simulink model "c6_formation2"  (R2021b)
settings: Solver=FixedStepDiscrete  StartTime=0.0  StopTime=Inf  FixedStep=sampleTime  RelTol=1e-3  EnableMultiTasking=on
PreLoadFcn:
  | %load emptyMap
  | 
  | % Lidar parameters
  | sensorOffset = [0,0];
  | scanAngles = -pi:pi/6:pi;
  | maxRange = 0.25;
InitFcn:
  | sampleTime = 0.05;
  | nMedianSize=3;
  | % Robot parameters
  | wheelRadius = 0.0335;
  | robotRadius = 0.7*0.116;
  | 
  | %角速度坐标
  | ks=1;
  | 
  | % Lidar parameters
  | sensorOffset = [0,0];
  | scanAngles = -pi:pi/36:pi;
  | maxRange = 0.2;
  | 
  | %车初始位置
  | init_pose_1=[1  1.3  pi/2]';
  | init_pose_2=[0.85 1  pi/2]';
  | init_pose_3=[1.15 1  pi/2]';
  | init_pose_4=[0.7  0.7 pi/2]';
  | init_pose_5=[1  0.7 pi/2]';
  | init_pose_6=[1.3 0.7  pi/2]';
  | 
  | %pp算法性能参数
  | Vd_pp=0.25;
  | Wd_pp=0.25*pi;
  | dist_pp=0.2;
  | GoalRadius=0.1;
  | numSector=72;
  | rangeDis=[0.03,maxRange];
  | thresholds=[0.03 0.1];
  | safetyDis=0.1;
  | minimumTurningRadius=0.2*0.2/3;
undefined symbols (not defined in the file): Angular, DiscIntNeverNeededParam, Linear, recovery_w
libraries: robotlib x24, dspstat3 x18, robotalgslib x6
(part 4 of 4)

== matlab function c6_formation2/controller/Car6/ppCar/Compute Velocity and Heading for Path following/Car1/Kinematicc Controller/MATLAB Function ==
  data: psi input; dw output; psid input; x input; xd input; y input; yd input; targetdir output
function [dw,targetdir]= fcn(psi,psid,x,xd,y,yd)

if norm([xd-x,yd-y])<0.15    
    targetdir=angdiff(psi,psid);
    dw=tanh(targetdir);    
else
    dw=0;
    targetdir=angdiff(psi,atan2(yd-y,xd-x));
end

== matlab function c6_formation2/controller/controller1/MATLAB Function5 ==
  data: poses input; idx input; ranges output; maxRange parameter; scanAngles parameter; robotRadius parameter

function ranges = genLidarSensor(poses,idx, maxRange, scanAngles, robotRadius)
%模拟激光雷达计算地图中障碍物距离

%计算部分
map=occupancyMap(3,3,50);
num=length(poses(1,:));%机器人总数
worldOffset=[0.5,0.5];%将世界坐标系偏移进地图
safetyDis=maxRange;
poseX=[poses(1,:)+worldOffset(1);poses(2,:)+worldOffset(2);poses(3,:)];
% for i=[1:idx-1 idx+1:num]
%     if poseX(i,1)>=0&&poseX(i,1)<=3&&poseX(i,2)>=0&&poseX(i,2)<=3        
%         setOccupancy(map,poseX(1:2,i)',1);
%     end
% end
obstacles = poseX(1:2,[1:idx-1 idx+1:num])';
setOccupancy(map,obstacles,ones(length(obstacles),1));
inflate(map,robotRadius);

if poseX(1,idx)>=0&&poseX(1,idx)<=3&&poseX(2,idx)>=0&&poseX(2,idx)<=3 
    vehiclePose = poseX(:,idx)';
    intsectionPts = rayIntersection(map,vehiclePose,scanAngles,safetyDis,0.7);
    offsets=intsectionPts-ones(length(scanAngles),1)*vehiclePose(1:2);
    ranges = sqrt(sum(offsets.^2,2));    
else
    ranges = nan(length(scanAngles),1);   
end

== matlab function c6_formation2/Subsystem/Car Pose Listener3/Subsystem/sensor2vCar4 ==
  data: V output; W output; VW_New input; VW_Msg input
function [V,W] = sensor2vCar(VW_New, VW_Msg)
persistent v0 w0
if isempty(v0)
    v0=0; 
    w0=0;    
end
if VW_New
    v0=VW_Msg.Linear.X;
    w0=VW_Msg.Angular.Z;
end

V=v0;
W=-w0;

== stateflow chart c6_formation2/Chart ==
  state Init
    %初始化各变量，第一批航路点
    state=1;
    wp=[1,1.3,pi/2;0.85,1,pi/2;1.15,1,pi/2;0.7,0.7,pi/2;1,0.7,pi/2;1.3,0.7,pi/2];
  state DuiXingBianHuan
    state SanKai
      %散开到一边[4 2 1 3 6;5]
      [wp,state]=s1_ComputeDist(poses);
    state LieDui
      %散开一遍到顺序另一边【6；5 4  3 2 1】
      [wp,state]=s2_ComputeDist(poses);
    state FengCao
      %聚到一起的蜂巢形[1;2 3; 4 5 6]，
      [wp,state]=s5_ComputeDist(poses);
    state Circle
      %绕中心画圈
      [wp,state]=s3_ComputeDist(poses);
    state DuiDao
      %从[1 2 3; 4 5 6]，对倒到【6 5 4；3 2 1】
      [wp,state]=s4_ComputeDist(poses);
    state default
    state LiuBianXing
      %六边形循环
      [wp,state]=s6_ComputeDist(poses);
    state TanChiShe
      %贪吃蛇循环
      [wp,state]=s7_ComputeDist(poses);
    DuiXingBianHuan -> SanKai [order 1] : [state==1]
    DuiXingBianHuan -> LieDui [order 2] : [state==2]
    DuiXingBianHuan -> FengCao [order 6] : [state==5]
    DuiXingBianHuan -> Circle [order 5] : [state==3]
    (default) -> default
    DuiXingBianHuan -> DuiDao [order 4] : [state==4]
    DuiXingBianHuan -> LiuBianXing [order 3] : [state==6]
    DuiXingBianHuan -> TanChiShe [order 7] : [state==7]
  (default) -> Init
  Init -> DuiXingBianHuan
  data: pose10 function_input; wp1 function_output; state2 function_output; pose10 function_input; wp1 function_output; state2 function_output; pose10 function_input; wp1 function_output; state2 function_output; pose10 function_input; wp1 function_output; state2 function_output; pose10 function_input; wp1 function_output; state2 function_output; pose10 function_input; wp1 function_output; state2 function_output; pose10 function_input; wp1 function_output; state2 function_output; wp output; poses input; state local
  function [wp1,state2]=s1_ComputeDist(pose10):
    | function [wp1,state2]=s1_ComputeDist(pose10)
    |     flag=zeros(6,1);
    |     wpSanKai=[1,1.8,pi/2;0.6,1.8,pi/2;1.4,1.8,pi/2;0.2,1.8,pi/2;1,1.4,pi/2;1.8,1.8,pi/2];
    |     wp1=wpSanKai;
    |     
    |     pos1=pose10(1,1:2);
    |     pos2=pose10(2,1:2);
    |     pos3=pose10(3,1:2);
    |     pos4=pose10(4,1:2);
    |     pos5=pose10(5,1:2);
    |     pos6=pose10(6,1:2);    
    |     dis_end=0.15;ang_end=30/180*pi;
    | 
    |     if norm(wp1(1,1:2)-pos1)<dis_end
    |         wp1(1,1:2)=pos1;
    |         if abs(angdiff(wp1(1,3),pose10(1,3)))<ang_end
    |             flag(1)=1;     
    |         end
    |     end
    |     if norm(wp1(2,1:2)-pos2)<dis_end
    |         wp1(2,1:2)=pos2;
    |         if abs(angdiff(wp1(2,3),pose10(2,3)))<ang_end
    |             flag(2)=1;     
    |         end        
    |     end
    |     if norm(wp1(3,1:2)-pos3)<dis_end
    |         wp1(3,1:2)=pos3;
    |         if abs(angdiff(wp1(3,3),pose10(3,3)))<ang_end
    |             flag(3)=1;     
    |         end  
    |     end
    |     if norm(wp1(4,1:2)-pos4)<dis_end
    |         wp1(4,1:2)=pos4;
    |         if abs(angdiff(wp1(4,3),pose10(4,3)))<ang_end
    |             flag(4)=1;     
    |         end  
    |     end
    |     if norm(wp1(5,1:2)-pos5)<dis_end
    |         wp1(5,1:2)=pos5;
    |         if abs(angdiff(wp1(5,3),pose10(5,3)))<ang_end
    |             flag(5)=1;     
    |         end  
    |     end
    |     if norm(wp1(6,1:2)-pos6)<dis_end
    |         wp1(6,1:2)=pos6;
    |         if abs(angdiff(wp1(6,3),pose10(6,3)))<ang_end
    |             flag(6)=1;     
    |         end  
    |     end
    |     
    |     if sum(flag)==6
    |         state2=2;
    |     else
    |         state2=1;
    |     end
    | end
  function [wp1,state2]=s2_ComputeDist(pose10):
    | function [wp1,state2]=s2_ComputeDist(pose10)
    |     flag=zeros(6,1);
    |     wplieDui=[1.8,0.2,0;1.4,0.2,-pi/2;1,0.2,-pi/2;0.6,0.2,-pi/2;0.2,0.2,-pi/2;0.2,0.6,-pi/2];
    |     wp1=wplieDui;
    |     
    |     pos1=pose10(1,1:2);
    |     pos2=pose10(2,1:2);
    |     pos3=pose10(3,1:2);
    |     pos4=pose10(4,1:2);
    |     pos5=pose10(5,1:2);
    |     pos6=pose10(6,1:2);    
    |     dis_end=0.15;ang_end=30/180*pi;
    |     
    |      if norm(wp1(1,1:2)-pos1)<dis_end
    |         wp1(1,1:2)=pos1;
    |         if abs(angdiff(wp1(1,3),pose10(1,3)))<ang_end
    |             flag(1)=1;     
    |         end
    |     end
    |     if norm(wp1(2,1:2)-pos2)<dis_end
    |         wp1(2,1:2)=pos2;
    |         if abs(angdiff(wp1(2,3),pose10(2,3)))<ang_end
    |             flag(2)=1;     
    |         end        
    |     end
    |     if norm(wp1(3,1:2)-pos3)<dis_end
    |         wp1(3,1:2)=pos3;
    |         if abs(angdiff(wp1(3,3),pose10(3,3)))<ang_end
    |             flag(3)=1;     
    |         end  
    |     end
    |     if norm(wp1(4,1:2)-pos4)<dis_end
    |         wp1(4,1:2)=pos4;
    |         if abs(angdiff(wp1(4,3),pose10(4,3)))<ang_end
    |             flag(4)=1;     
    |         end  
    |     end
    |     if norm(wp1(5,1:2)-pos5)<dis_end
    |         wp1(5,1:2)=pos5;
    |         if abs(angdiff(wp1(5,3),pose10(5,3)))<ang_end
    |             flag(5)=1;     
    |         end  
    |     end
    |     if norm(wp1(6,1:2)-pos6)<dis_end
    |         wp1(6,1:2)=pos6;
    |         if abs(angdiff(wp1(6,3),pose10(6,3)))<5/180*pi
    |             flag(6)=1;     
    |         end  
    |     end
    |     
    |     if sum(flag)==6
    |         state2=3;
    |     else
    |         state2=2;
    |     end
    | end
  function [wp1,state2]=s3_ComputeDist(pose10):
    | function [wp1,state2]=s3_ComputeDist(pose10)
    |     persistent idx inum istart
    |     if isempty(idx)
    |         idx=2;%转圈标识,初始值根据实际效果调整
    |         inum=1;%转几圈标识
    |         istart=0;%转圈前排队
    |     end
    |     flag=zeros(6,1);
    |     wp1=pose10;
    |     t=(0:30:330)/180*pi;x=1+0.8*cos(t);y=1+0.8*sin(t);
    |     wpCircle=[x;y;t+pi/2]';    
    |     
    |     switch idx
    |         case 1
    |             wp1(1:6,:)=[wpCircle(idx,:);wpCircle(end:-1:end-4,:)];
    |         case 2
    |             wp1(1:6,:)=[wpCircle(idx:-1:1,:);wpCircle(end:-1:end-3,:)];
    |         case 3
    |             wp1(1:6,:)=[wpCircle(idx:-1:1,:);wpCircle(end:-1:end-2,:)];
    |         case 4
    |             wp1(1:6,:)=[wpCircle(idx:-1:1,:);wpCircle(end:-1:end-1,:)];
    |         case 5
    |             wp1(1:6,:)=[wpCircle(idx:-1:1,:);wpCircle(end,:)];
    |         otherwise
    |            wp1(1:6,:)=wpCircle(idx:-1:idx-5,:);
    |     end
    |     
    |     pos1=pose10(1,1:2);
    |     pos2=pose10(2,1:2);
    |     pos3=pose10(3,1:2);
    |     pos4=pose10(4,1:2);
    |     pos5=pose10(5,1:2);
    |     pos6=pose10(6,1:2);
    |     dis_end=0.15;ang_end=30/180*pi;
    |     
    |     if norm(wp1(1,1:2)-pos1)<dis_end
    |         wp1(1,1:2)=pos1;
    |         
    |         if ~istart&&abs(angdiff(wp1(1,3),pose10(1,3)))<ang_end
    |             flag(1)=1;          
    |         end   
    |         if istart       
    |             idx=idx+1;
    |         end
    |         if idx>length(wpCircle(:,1))
    |             idx=1;
    |             inum=inum+1;
    |         end
    |     end
    | 
    |      if norm(wp1(2,1:2)-pos2)<dis_end
    |         wp1(2,1:2)=pos2;
    |         if abs(angdiff(wp1(2,3),pose10(2,3)))<ang_end
    |             flag(2)=1;     
    |         end        
    |     end
    |     if norm(wp1(3,1:2)-pos3)<dis_end
    |         wp1(3,1:2)=pos3;
    |         if abs(angdiff(wp1(3,3),pose10(3,3)))<ang_end
    |             flag(3)=1;     
    |         end  
    |     end
    |     if norm(wp1(4,1:2)-pos4)<dis_end
    |         wp1(4,1:2)=pos4;
    |         if abs(angdiff(wp1(4,3),pose10(4,3)))<ang_end
    |             flag(4)=1;     
    |         end  
    |     end
    |     if norm(wp1(5,1:2)-pos5)<dis_end
    |         wp1(5,1:2)=pos5;
    |         if abs(angdiff(wp1(5,3),pose10(5,3)))<ang_end
    |             flag(5)=1;     
    |         end  
    |     end
    |     if norm(wp1(6,1:2)-pos6)<dis_end
    |         wp1(6,1:2)=pos6;
    |         if abs(angdiff(wp1(6,3),pose10(6,3)))<ang_end
    |             flag(6)=1;     
    |         end  
    |     end
    | 
    |  %转圈前先排好位置
    |  if ~istart
    |     if sum(flag)==6
    |         istart=1;        
    |     end 
    |  end
    |     
    | 
    | if inum==2&&idx==6
    |     state2=7;
    |     idx=2;inum=1;istart=0;%离开该状态前需要复位
    | else
    |     state2=3;
    | end
  function [wp1,state2]=s4_ComputeDist(pose10):
    | function [wp1,state2]=s4_ComputeDist(pose10)
    |     persistent inum iflag
    |     if isempty(inum)
    |         inum=1;%对倒次数计数
    |         iflag=2;%上下状态标识
    |     end
    |     flag=zeros(6,1);
    |     wpDuiDao1=[0.2,1.8,pi;1,1.8,pi;1.8,1.8,pi;0.2,0.2,0;1,0.2,0;1.8,0.2,0];
    |     wpDuiDao2=[0.6,0.6,-pi/2;0.8,1,-pi/2;1,1.4,-pi/2;1,0.6,pi/2;1.2,1,pi/2;1.4,1.4,pi/2];
    |     wpDuiDao3=[1.8,0.2,0;1,0.2,0;0.2,0.2,0;1.8,1.8,-pi;1,1.8,-pi;0.2,1.8,-pi];
    |     wpDuiDao4=[1.4,1.4,pi/2;1.2,1,pi/2;1,0.6,pi/2;1,1.4,-pi/2;0.8,1,-pi/2;0.6,0.6,-pi/2];
    |     switch iflag
    |         case 0
    |             wp1=wpDuiDao1;
    |         case 1
    |             wp1=wpDuiDao2;
    |         case 2
    |             wp1=wpDuiDao3;
    |         otherwise
    |             wp1=wpDuiDao4;
    |     end    
    |     pos1=pose10(1,1:2);
    |     pos2=pose10(2,1:2);
    |     pos3=pose10(3,1:2);
    |     pos4=pose10(4,1:2);
    |     pos5=pose10(5,1:2);
    |     pos6=pose10(6,1:2); 
    |     dis_end=0.15;ang_end=30/180*pi;
    |             
    |     %首先判断是否到达目的地
    |      if norm(wp1(1,1:2)-pos1)<dis_end
    |         wp1(1,1:2)=pos1;
    |         if abs(angdiff(wp1(1,3),pose10(1,3)))<ang_end
    |             flag(1)=1;     
    |         end
    |     end
    |     if norm(wp1(2,1:2)-pos2)<dis_end
    |         wp1(2,1:2)=pos2;
    |         if abs(angdiff(wp1(2,3),pose10(2,3)))<ang_end
    |             flag(2)=1;     
    |         end        
    |     end
    |     if norm(wp1(3,1:2)-pos3)<dis_end
    |         wp1(3,1:2)=pos3;
    |         if abs(angdiff(wp1(3,3),pose10(3,3)))<ang_end
    |             flag(3)=1;     
    |         end  
    |     end
    |     if norm(wp1(4,1:2)-pos4)<dis_end
    |         wp1(4,1:2)=pos4;
    |         if abs(angdiff(wp1(4,3),pose10(4,3)))<ang_end
    |             flag(4)=1;     
    |         end  
    |     end
    |     if norm(wp1(5,1:2)-pos5)<dis_end
    |         wp1(5,1:2)=pos5;
    |         if abs(angdiff(wp1(5,3),pose10(5,3)))<ang_end
    |             flag(5)=1;     
    |         end  
    |     end
    |     if norm(wp1(6,1:2)-pos6)<dis_end
    |         wp1(6,1:2)=pos6;
    |         if abs(angdiff(wp1(6,3),pose10(6,3)))<5/180*pi
    |             flag(6)=1;     
    |         end  
    |     end
    |    
    |     if sum(flag)==6     
    |         iflag=iflag+1;
    |         if iflag>3
    |             iflag=0;
    |             inum=inum+1; 
    |         end        
    |     end
    |     if inum==3&&iflag==1
    |         state2=5;
    |         inum=1;iflag=2;%离开前复位
    |     else
    |         state2=4;
    |     end
    | end
  function [wp1,state2]=s5_ComputeDist(pose10):
    | function [wp1,state2]=s5_ComputeDist(pose10)
    |     persistent st
    |     if isempty(st)
    |         st=0;
    |     end
    |     flag=zeros(6,1);
    |     wpFengChao=[1,1.3,pi/2;0.85,1,pi;1.15,1,0;0.7,0.7,pi/2;1,0.7,pi/2;1.3,0.7,pi/2];
    |     wp1=wpFengChao;
    |     
    |     pos1=pose10(1,1:2);
    |     pos2=pose10(2,1:2);
    |     pos3=pose10(3,1:2);
    |     pos4=pose10(4,1:2);
    |     pos5=pose10(5,1:2);
    |     pos6=pose10(6,1:2);    
    |     dis_end=0.15;ang_end=30/180*pi;
    |     
    |      if norm(wp1(1,1:2)-pos1)<dis_end
    |         wp1(1,1:2)=pos1;
    |         if abs(angdiff(wp1(1,3),pose10(1,3)))<ang_end
    |             flag(1)=1;     
    |         end
    |     end
    |     if norm(wp1(2,1:2)-pos2)<dis_end
    |         wp1(2,1:2)=pos2;
    |         if abs(angdiff(wp1(2,3),pose10(2,3)))<ang_end
    |             flag(2)=1;     
    |         end        
    |     end
    |     if norm(wp1(3,1:2)-pos3)<dis_end
    |         wp1(3,1:2)=pos3;
    |         if abs(angdiff(wp1(3,3),pose10(3,3)))<ang_end
    |             flag(3)=1;     
    |         end  
    |     end
    |     if norm(wp1(4,1:2)-pos4)<dis_end
    |         wp1(4,1:2)=pos4;
    |         if abs(angdiff(wp1(4,3),pose10(4,3)))<ang_end
    |             flag(4)=1;     
    |         end  
    |     end
    |     if norm(wp1(5,1:2)-pos5)<dis_end
    |         wp1(5,1:2)=pos5;
    |         if abs(angdiff(wp1(5,3),pose10(5,3)))<ang_end
    |             flag(5)=1;     
    |         end  
    |     end
    |     if norm(wp1(6,1:2)-pos6)<dis_end
    |         wp1(6,1:2)=pos6;
    |         if abs(angdiff(wp1(6,3),pose10(6,3)))<ang_end
    |             flag(6)=1;     
    |         end  
    |     end
    |     
    |     if sum(flag)==6
    |         if st>5
    |             st=0;%重新开始前暂停5s
    |             state2=1;
    |         else
    |             st=st+0.05;
    |             state2=5;
    |         end
    |     else
    |         state2=5;
    |     end
    | end
  function [wp1,state2]=s6_ComputeDist(pose10):
    | function [wp1,state2]=s6_ComputeDist(pose10)
    |     persistent idx inum istart
    |     if isempty(idx)
    |         idx=1;%转圈标识,初始值根据实际效果调整
    |         inum=1;%转几圈标识
    |         istart=0;%转圈前排队
    |     end
    |     flag=zeros(6,1);
    |     wp1=pose10;
    |     wpLiuBianXing=[1,1.8,0;1-0.8*sin(pi/3),1+0.8*cos(pi/3),pi/3;1-0.8*sin(pi/3),1-0.8*cos(pi/3),pi*2/3;...
    |               1,0.2,pi;1+0.8*sin(pi/3),1-0.8*cos(pi/3),-pi*2/3;1+0.8*sin(pi/3),1+0.8*cos(pi/3),-pi/3];    
    |     
    |     switch idx
    |         case 1
    |             wp1(1:6,:)=wpLiuBianXing(1:6,:);
    |         case 2
    |             wp1(1:6,:)=wpLiuBianXing([2:6,1],:);
    |         case 3
    |             wp1(1:6,:)=wpLiuBianXing([3:6,1:2],:);
    |         case 4
    |             wp1(1:6,:)=wpLiuBianXing([4:6,1:3],:);
    |         case 5
    |             wp1(1:6,:)=wpLiuBianXing([5:6,1:4],:);
    |         otherwise
    |            wp1(1:6,:)=wpLiuBianXing([6,1:5],:);
    |     end
    |     
    |     pos1=pose10(1,1:2);
    |     pos2=pose10(2,1:2);
    |     pos3=pose10(3,1:2);
    |     pos4=pose10(4,1:2);
    |     pos5=pose10(5,1:2);
    |     pos6=pose10(6,1:2);
    |     dis_end=0.15;ang_end=30/180*pi;
    |     
    |     if norm(wp1(1,1:2)-pos1)<dis_end
    |         wp1(1,1:2)=pos1;
    |         
    |         if ~istart&&abs(angdiff(wp1(1,3),pose10(1,3)))<ang_end
    |             flag(1)=1;          
    |         end   
    |         if istart       
    |             idx=idx-1;
    |         end
    |         if idx<1
    |             idx=length(wpLiuBianXing(:,1));
    |             inum=inum+1;
    |         end
    |     end
    | 
    |      if norm(wp1(2,1:2)-pos2)<dis_end
    |         wp1(2,1:2)=pos2;
    |         if abs(angdiff(wp1(2,3),pose10(2,3)))<ang_end
    |             flag(2)=1;     
    |         end        
    |     end
    |     if norm(wp1(3,1:2)-pos3)<dis_end
    |         wp1(3,1:2)=pos3;
    |         if abs(angdiff(wp1(3,3),pose10(3,3)))<ang_end
    |             flag(3)=1;     
    |         end  
    |     end
    |     if norm(wp1(4,1:2)-pos4)<dis_end
    |         wp1(4,1:2)=pos4;
    |         if abs(angdiff(wp1(4,3),pose10(4,3)))<ang_end
    |             flag(4)=1;     
    |         end  
    |     end
    |     if norm(wp1(5,1:2)-pos5)<dis_end
    |         wp1(5,1:2)=pos5;
    |         if abs(angdiff(wp1(5,3),pose10(5,3)))<ang_end
    |             flag(5)=1;     
    |         end  
    |     end
    |     if norm(wp1(6,1:2)-pos6)<dis_end
    |         wp1(6,1:2)=pos6;
    |         if abs(angdiff(wp1(6,3),pose10(6,3)))<ang_end
    |             flag(6)=1;     
    |         end  
    |     end
    | 
    |  %转圈前先排好位置
    |  if ~istart
    |     if sum(flag)==6
    |         istart=1;        
    |     end 
    |  end
    |     
    | 
    | if inum>1&&idx<2
    |     state2=4;
    |     idx=1;inum=1;istart=0;%离开该状态前需要复位
    | else
    |     state2=6;
    | end
  function [wp1,state2]=s7_ComputeDist(pose10):
    | function [wp1,state2]=s7_ComputeDist(pose10)
    |     %此版本检测超时5s不动，判断为卡住，进入下一状态
    |     persistent pos10 t0
    |     if isempty(pos10)
    |         pos10=nan(6,2);
    |         t0=0;
    |     end    
    |     persistent idx inum istart
    |     if isempty(idx)
    |         idx=18;%转圈标识,初始值根据实际效果调整
    |         inum=1;%转几圈标识
    |         istart=0;%转圈前排队
    |     end
    |     flag=zeros(6,1);
    |     wp1=pose10;    
    |     wpTanchishe=[[linspace(0.2,1.8,4);linspace(0.2,0.2,4);linspace(0,0,4)]';[linspace(1.8,0.2,4);linspace(0.73,0.73,4);linspace(pi,pi,4)]';...
    |                  [linspace(0.2,1.8,4);linspace(1.27,1.27,4);linspace(0,0,4)]';[linspace(1.8,0.2,4);linspace(1.8,1.8,4);linspace(pi,pi,4)]';...                      
    |                  [linspace(0.2,0.2,2);linspace(1.27,0.73,2);linspace(-pi/2,-pi/2,2)]'];    %弓字形
    |     
    |     switch idx
    |         case 1
    |             wp1(1:6,:)=[wpTanchishe(idx,:);wpTanchishe(end:-1:end-4,:)];
    |         case 2
    |             wp1(1:6,:)=[wpTanchishe(idx:-1:1,:);wpTanchishe(end:-1:end-3,:)];
    |         case 3
    |             wp1(1:6,:)=[wpTanchishe(idx:-1:1,:);wpTanchishe(end:-1:end-2,:)];
    |         case 4
    |             wp1(1:6,:)=[wpTanchishe(idx:-1:1,:);wpTanchishe(end:-1:end-1,:)];
    |         case 5
    |             wp1(1:6,:)=[wpTanchishe(idx:-1:1,:);wpTanchishe(end,:)];
    |         otherwise
    |            wp1(1:6,:)=wpTanchishe(idx:-1:idx-5,:);
    |     end
    |     
    |     pos1=pose10(1,1:2);
    |     pos2=pose10(2,1:2);
    |     pos3=pose10(3,1:2);
    |     pos4=pose10(4,1:2);
    |     pos5=pose10(5,1:2);
    |     pos6=pose10(6,1:2);
    |     dis_end=0.12;ang_end=15/180*pi;
    |     
    |     if norm(wp1(1,1:2)-pos1)<dis_end
    |         wp1(1,1:2)=pos1;
    |         
    |         if ~istart&&abs(angdiff(wp1(1,3),pose10(1,3)))<ang_end
    |             flag(1)=1;          
    |         end   
    |         if istart       
    |             idx=idx+1;
    |         end
    |         if idx>length(wpTanchishe(:,1))
    |             idx=1;
    |             inum=inum+1;
    |         end
    |     end
    | 
    |      if norm(wp1(2,1:2)-pos2)<dis_end
    |         wp1(2,1:2)=pos2;
    |         if abs(angdiff(wp1(2,3),pose10(2,3)))<ang_end
    |             flag(2)=1;     
    |         end        
    |     end
    |     if norm(wp1(3,1:2)-pos3)<0.1
    |         wp1(3,1:2)=pos3;
    |         if abs(angdiff(wp1(3,3),pose10(3,3)))<ang_end
    |             flag(3)=1;     
    |         end  
    |     end
    |     if norm(wp1(4,1:2)-pos4)<dis_end
    |         wp1(4,1:2)=pos4;
    |         if abs(angdiff(wp1(4,3),pose10(4,3)))<ang_end
    |             flag(4)=1;     
    |         end  
    |     end
    |     if norm(wp1(5,1:2)-pos5)<dis_end
    |         wp1(5,1:2)=pos5;
    |         if abs(angdiff(wp1(5,3),pose10(5,3)))<ang_end
    |             flag(5)=1;     
    |         end  
    |     end
    |     if norm(wp1(6,1:2)-pos6)<dis_end
    |         wp1(6,1:2)=pos6;
    |         if abs(angdiff(wp1(6,3),pose10(6,3)))<ang_end
    |             flag(6)=1;     
    |         end  
    |     end
    |     
    |     %防卡
    |     if norm(pos10(1,:)-pos1)<0.03&&norm(pos10(2,:)-pos2)<0.03...
    |             &&norm(pos10(3,:)-pos3)<0.03&&norm(pos10(4,:)-pos4)<0.03...
    |             &&norm(pos10(5,:)-pos5)<0.03&&norm(pos10(6,:)-pos6)<0.03
    |         t0=t0+0.05;
    |         if t0>5
    |             flag=ones(6,1);
    |         end
    |     else
    |         pos10=pose10(1:6,1:2);t0=0;
    |     end
    | 
    |      %转圈前先排好位置
    |      if ~istart
    |         if sum(flag)==6
    |             istart=1;        
    |         end 
    |      end
    |         
    |     
    |     if inum>2&&idx>10
    |         state2=6;
    |         idx=1;inum=1;istart=0;%离开该状态前需要复位
    |         pos10=nan(6,2); t0=0;
    |     else
    |         state2=7;
    |     end

== matlab function c6_formation2/Subsystem/Car Pose Listener4/Subsystem/sensor2vCar ==
  data: x_init output; y_init output; yaw_init output; flag output; poseNew input; poseMsg input
function [x_init,y_init,yaw_init,flag] = sensor2vCar(poseNew, poseMsg)
persistent x0 y0 yaw0 yaw1 x0_init y0_init yaw0_init fStart
if isempty(x0)
    x0=-10; y0=-10; yaw0=0; yaw1=0;   
    x0_init=-10;y0_init=-10;yaw0_init=0;
    fStart=0;
end
if poseNew
    if x0==poseMsg.Pose.Pose.Position.X&&y0==poseMsg.Pose.Pose.Position.Y
        flag=1;
    else
        x0=poseMsg.Pose.Pose.Position.X;
        y0=poseMsg.Pose.Pose.Position.Y;   
        %yaw2=atan2(2*(poseMsg.Pose.Pose.Orientation.Z*poseMsg.Pose.Pose.Orientation.W),1-2*(poseMsg.Pose.Pose.Orientation.Z^2)); 
        eul=quat2eul([poseMsg.Pose.Pose.Orientation.W,poseMsg.Pose.Pose.Orientation.X,poseMsg.Pose.Pose.Orientation.Y,poseMsg.Pose.Pose.Orientation.Z]);
        yaw2=eul(1);
        %对前后角度差使用积分，恢复yaw的连续性
        yaw0=yaw0+angdiff(yaw1,yaw2);
        yaw1=yaw2;
        flag=0;        
        x0_init=x0;
        y0_init=y0;
        yaw0_init=yaw0;
        fStart=1;
    end 
else
    if fStart
        flag=1;
    else
        flag=0;
    end
end

x_init=x0_init;y_init=y0_init;yaw_init=yaw0_init;

== matlab function c6_formation2/Subsystem/Car Pose Listener4/Subsystem/sensor2vCar4 ==
  data: V output; W output; VW_New input; VW_Msg input
function [V,W] = sensor2vCar(VW_New, VW_Msg)
persistent v0 w0
if isempty(v0)
    v0=0; 
    w0=0;    
end
if VW_New
    v0=VW_Msg.Linear.X;
    w0=VW_Msg.Angular.Z;
end

V=v0;
W=-w0;

== matlab function c6_formation2/Subsystem/Car Pose Listener5/Subsystem/sensor2vCar ==
  data: x_init output; y_init output; yaw_init output; flag output; poseNew input; poseMsg input
function [x_init,y_init,yaw_init,flag] = sensor2vCar(poseNew, poseMsg)
persistent x0 y0 yaw0 yaw1 x0_init y0_init yaw0_init fStart
if isempty(x0)
    x0=-10; y0=-10; yaw0=0; yaw1=0;   
    x0_init=-10;y0_init=-10;yaw0_init=0;
    fStart=0;
end
if poseNew
    if x0==poseMsg.Pose.Pose.Position.X&&y0==poseMsg.Pose.Pose.Position.Y
        flag=1;
    else
        x0=poseMsg.Pose.Pose.Position.X;
        y0=poseMsg.Pose.Pose.Position.Y;   
        %yaw2=atan2(2*(poseMsg.Pose.Pose.Orientation.Z*poseMsg.Pose.Pose.Orientation.W),1-2*(poseMsg.Pose.Pose.Orientation.Z^2)); 
        eul=quat2eul([poseMsg.Pose.Pose.Orientation.W,poseMsg.Pose.Pose.Orientation.X,poseMsg.Pose.Pose.Orientation.Y,poseMsg.Pose.Pose.Orientation.Z]);
        yaw2=eul(1);
        %对前后角度差使用积分，恢复yaw的连续性
        yaw0=yaw0+angdiff(yaw1,yaw2);
        yaw1=yaw2;
        flag=0;        
        x0_init=x0;
        y0_init=y0;
        yaw0_init=yaw0;
        fStart=1;
    end 
else
    if fStart
        flag=1;
    else
        flag=0;
    end
end

x_init=x0_init;y_init=y0_init;yaw_init=yaw0_init;

== matlab function c6_formation2/Subsystem/Car Pose Listener5/Subsystem/sensor2vCar4 ==
  data: V output; W output; VW_New input; VW_Msg input
function [V,W] = sensor2vCar(VW_New, VW_Msg)
persistent v0 w0
if isempty(v0)
    v0=0; 
    w0=0;    
end
if VW_New
    v0=VW_Msg.Linear.X;
    w0=VW_Msg.Angular.Z;
end

V=v0;
W=-w0;

== matlab function c6_formation2/controller/controller1/MATLAB Function2 ==
  data: poses input; idx input; ranges output; maxRange parameter; scanAngles parameter; robotRadius parameter

function ranges = genLidarSensor(poses,idx, maxRange, scanAngles, robotRadius)
%模拟激光雷达计算地图中障碍物距离

%计算部分
map=occupancyMap(3,3,50);
num=length(poses(1,:));%机器人总数
worldOffset=[0.5,0.5];%将世界坐标系偏移进地图
safetyDis=maxRange;
poseX=[poses(1,:)+worldOffset(1);poses(2,:)+worldOffset(2);poses(3,:)];
% for i=[1:idx-1 idx+1:num]
%     if poseX(i,1)>=0&&poseX(i,1)<=3&&poseX(i,2)>=0&&poseX(i,2)<=3        
%         setOccupancy(map,poseX(1:2,i)',1);
%     end
% end
obstacles = poseX(1:2,[1:idx-1 idx+1:num])';
setOccupancy(map,obstacles,ones(length(obstacles),1));
inflate(map,robotRadius);

if poseX(1,idx)>=0&&poseX(1,idx)<=3&&poseX(2,idx)>=0&&poseX(2,idx)<=3 
    vehiclePose = poseX(:,idx)';
    intsectionPts = rayIntersection(map,vehiclePose,scanAngles,safetyDis,0.7);
    offsets=intsectionPts-ones(length(scanAngles),1)*vehiclePose(1:2);
    ranges = sqrt(sum(offsets.^2,2));    
else
    ranges = nan(length(scanAngles),1);   
end

== matlab function c6_formation2/controller/controller1/MATLAB Function3 ==
  data: poses input; idx input; ranges output; maxRange parameter; scanAngles parameter; robotRadius parameter

function ranges = genLidarSensor(poses,idx, maxRange, scanAngles, robotRadius)
%模拟激光雷达计算地图中障碍物距离

%计算部分
map=occupancyMap(3,3,50);
num=length(poses(1,:));%机器人总数
worldOffset=[0.5,0.5];%将世界坐标系偏移进地图
safetyDis=maxRange;
poseX=[poses(1,:)+worldOffset(1);poses(2,:)+worldOffset(2);poses(3,:)];
% for i=[1:idx-1 idx+1:num]
%     if poseX(i,1)>=0&&poseX(i,1)<=3&&poseX(i,2)>=0&&poseX(i,2)<=3        
%         setOccupancy(map,poseX(1:2,i)',1);
%     end
% end
obstacles = poseX(1:2,[1:idx-1 idx+1:num])';
setOccupancy(map,obstacles,ones(length(obstacles),1));
inflate(map,robotRadius);

if poseX(1,idx)>=0&&poseX(1,idx)<=3&&poseX(2,idx)>=0&&poseX(2,idx)<=3 
    vehiclePose = poseX(:,idx)';
    intsectionPts = rayIntersection(map,vehiclePose,scanAngles,safetyDis,0.7);
    offsets=intsectionPts-ones(length(scanAngles),1)*vehiclePose(1:2);
    ranges = sqrt(sum(offsets.^2,2));    
else
    ranges = nan(length(scanAngles),1);   
end

== matlab function c6_formation2/controller/controller1/MATLAB Function10 ==
  data: poses input; idx input; ranges output; maxRange parameter; scanAngles parameter; robotRadius parameter

function ranges = genLidarSensor(poses,idx, maxRange, scanAngles, robotRadius)
%模拟激光雷达计算地图中障碍物距离

%计算部分
map=occupancyMap(3,3,50);
num=length(poses(1,:));%机器人总数
worldOffset=[0.5,0.5];%将世界坐标系偏移进地图
safetyDis=maxRange;
poseX=[poses(1,:)+worldOffset(1);poses(2,:)+worldOffset(2);poses(3,:)];
% for i=[1:idx-1 idx+1:num]
%     if poseX(i,1)>=0&&poseX(i,1)<=3&&poseX(i,2)>=0&&poseX(i,2)<=3        
%         setOccupancy(map,poseX(1:2,i)',1);
%     end
% end
obstacles = poseX(1:2,[1:idx-1 idx+1:num])';
setOccupancy(map,obstacles,ones(length(obstacles),1));
inflate(map,robotRadius);

if poseX(1,idx)>=0&&poseX(1,idx)<=3&&poseX(2,idx)>=0&&poseX(2,idx)<=3 
    vehiclePose = poseX(:,idx)';
    intsectionPts = rayIntersection(map,vehiclePose,scanAngles,safetyDis,0.7);
    offsets=intsectionPts-ones(length(scanAngles),1)*vehiclePose(1:2);
    ranges = sqrt(sum(offsets.^2,2));    
else
    ranges = nan(length(scanAngles),1);   
end

== matlab function c6_formation2/controller/controller1/MATLAB Function4 ==
  data: poses input; idx input; ranges output; maxRange parameter; scanAngles parameter; robotRadius parameter

function ranges = genLidarSensor(poses,idx, maxRange, scanAngles, robotRadius)
%模拟激光雷达计算地图中障碍物距离

%计算部分
map=occupancyMap(3,3,50);
num=length(poses(1,:));%机器人总数
worldOffset=[0.5,0.5];%将世界坐标系偏移进地图
safetyDis=maxRange;
poseX=[poses(1,:)+worldOffset(1);poses(2,:)+worldOffset(2);poses(3,:)];
% for i=[1:idx-1 idx+1:num]
%     if poseX(i,1)>=0&&poseX(i,1)<=3&&poseX(i,2)>=0&&poseX(i,2)<=3        
%         setOccupancy(map,poseX(1:2,i)',1);
%     end
% end
obstacles = poseX(1:2,[1:idx-1 idx+1:num])';
setOccupancy(map,obstacles,ones(length(obstacles),1));
inflate(map,robotRadius);

if poseX(1,idx)>=0&&poseX(1,idx)<=3&&poseX(2,idx)>=0&&poseX(2,idx)<=3 
    vehiclePose = poseX(:,idx)';
    intsectionPts = rayIntersection(map,vehiclePose,scanAngles,safetyDis,0.7);
    offsets=intsectionPts-ones(length(scanAngles),1)*vehiclePose(1:2);
    ranges = sqrt(sum(offsets.^2,2));    
else
    ranges = nan(length(scanAngles),1);   
end

== matlab function c6_formation2/Subsystem/Car Pose Listener/Subsystem/sensor2vCar ==
  data: x_init output; y_init output; yaw_init output; flag output; poseNew input; poseMsg input
function [x_init,y_init,yaw_init,flag] = sensor2vCar(poseNew, poseMsg)
persistent x0 y0 yaw0 yaw1 x0_init y0_init yaw0_init fStart
if isempty(x0)
    x0=-10; y0=-10; yaw0=0; yaw1=0;   
    x0_init=-10;y0_init=-10;yaw0_init=0;
    fStart=0;
end
if poseNew
    if x0==poseMsg.Pose.Pose.Position.X&&y0==poseMsg.Pose.Pose.Position.Y
        flag=1;
    else
        x0=poseMsg.Pose.Pose.Position.X;
        y0=poseMsg.Pose.Pose.Position.Y;   
        %yaw2=atan2(2*(poseMsg.Pose.Pose.Orientation.Z*poseMsg.Pose.Pose.Orientation.W),1-2*(poseMsg.Pose.Pose.Orientation.Z^2)); 
        eul=quat2eul([poseMsg.Pose.Pose.Orientation.W,poseMsg.Pose.Pose.Orientation.X,poseMsg.Pose.Pose.Orientation.Y,poseMsg.Pose.Pose.Orientation.Z]);
        yaw2=eul(1);
        %对前后角度差使用积分，恢复yaw的连续性
        yaw0=yaw0+angdiff(yaw1,yaw2);
        yaw1=yaw2;
        flag=0;        
        x0_init=x0;
        y0_init=y0;
        yaw0_init=yaw0;
        fStart=1;
    end 
else
    if fStart
        flag=1;
    else
        flag=0;
    end
end

x_init=x0_init;y_init=y0_init;yaw_init=yaw0_init;

== matlab function c6_formation2/Subsystem/Car Pose Listener1/Subsystem/sensor2vCar4 ==
  data: V output; W output; VW_New input; VW_Msg input
function [V,W] = sensor2vCar(VW_New, VW_Msg)
persistent v0 w0
if isempty(v0)
    v0=0; 
    w0=0;    
end
if VW_New
    v0=VW_Msg.Linear.X;
    w0=VW_Msg.Angular.Z;
end

V=v0;
W=-w0;

== matlab function c6_formation2/Subsystem/Car Pose Listener2/Subsystem/sensor2vCar ==
  data: x_init output; y_init output; yaw_init output; flag output; poseNew input; poseMsg input
function [x_init,y_init,yaw_init,flag] = sensor2vCar(poseNew, poseMsg)
persistent x0 y0 yaw0 yaw1 x0_init y0_init yaw0_init fStart
if isempty(x0)
    x0=-10; y0=-10; yaw0=0; yaw1=0;   
    x0_init=-10;y0_init=-10;yaw0_init=0;
    fStart=0;
end
if poseNew
    if x0==poseMsg.Pose.Pose.Position.X&&y0==poseMsg.Pose.Pose.Position.Y
        flag=1;
    else
        x0=poseMsg.Pose.Pose.Position.X;
        y0=poseMsg.Pose.Pose.Position.Y;   
        %yaw2=atan2(2*(poseMsg.Pose.Pose.Orientation.Z*poseMsg.Pose.Pose.Orientation.W),1-2*(poseMsg.Pose.Pose.Orientation.Z^2)); 
        eul=quat2eul([poseMsg.Pose.Pose.Orientation.W,poseMsg.Pose.Pose.Orientation.X,poseMsg.Pose.Pose.Orientation.Y,poseMsg.Pose.Pose.Orientation.Z]);
        yaw2=eul(1);
        %对前后角度差使用积分，恢复yaw的连续性
        yaw0=yaw0+angdiff(yaw1,yaw2);
        yaw1=yaw2;
        flag=0;        
        x0_init=x0;
        y0_init=y0;
        yaw0_init=yaw0;
        fStart=1;
    end 
else
    if fStart
        flag=1;
    else
        flag=0;
    end
end

x_init=x0_init;y_init=y0_init;yaw_init=yaw0_init;
